simulink model "soc_opt5_compressed"  (R2026a)
settings: Solver=FixedStepDiscrete  StopTime=9  FixedStep=1
values from neighbouring files (symbols this model uses):
  compNet = s.bestNet    [build_simulink_model.m]    (also in save_slx.m; setup_and_open_slx.m; step2_simulink_sim.m)
libraries: dlconvfclib x2, dlsequencelib x2, dlactivationlib x1
Description:
  | SOC estimation: proj10_quant (neuronPCA 10%% + dlquantizer int8). 77.5%% Flash savings. MAE=9.50e-04 vs PyTorch. MATLAB R2026a.
settings Model: Creator=arkadiyturevskiy  LastModifiedBy=arkadiyturevskiy
settings HardwareCC: ProdLargestAtomicInteger=Long  ProdLargestAtomicFloat=Double  ProdHWDeviceType=ARM Compatible->ARM Cortex-M
settings RTWCC: SystemTargetFile=ert.tlc  PortableWordSizes=on  Description=Embedded Coder
settings ERTTargetCC: GenerateSampleERTMain=on

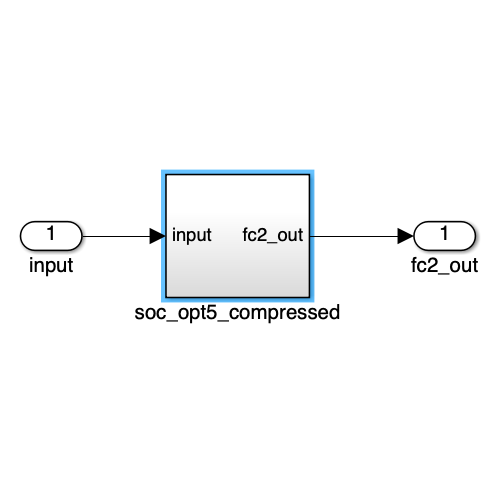
[thumbnail: Simulink's stored preview of the top-level diagram]
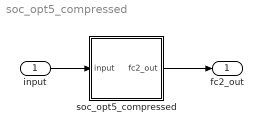
== system soc_opt5_compressed ==
  input : Inport  PortDimensions="[5  1]"
  soc_opt5_compressed : Subsystem
  fc2_out : Outport
  wires:
  soc_opt5_compressed/1(fc2_out) -> fc2_out/1
  input/1 -> soc_opt5_compressed/1(input)

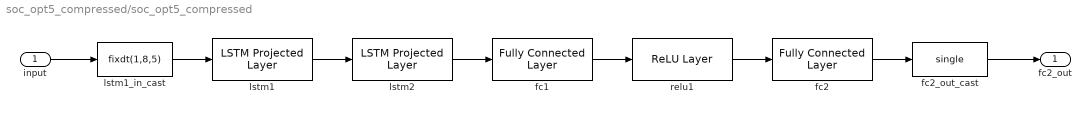
== system soc_opt5_compressed/soc_opt5_compressed ==
  input : Inport  PortDimensions="[5  1]"
  fc1 : dlconvfclib/Fully Connected Layer  Layer=compNet.Layers(4)  OutMin=[]  OutMax=[]  OutDataTypeStr=fixdt(1,8,7)  RndMeth=Nearest  SaturateOnIntegerOverflow=on  WeightsDataTypeStr=fixdt(1,8,10)  WeightsMin=[]  WeightsMax=[]  BiasDataTypeStr=fixdt(1,32,19)  BiasMin=[]  BiasMax=[]  AccumDataTypeStr=fixdt(1,32,19)  AccumMin=[]  AccumMax=[]  InternalRndMeth=Nearest  InternalSaturateOnIntegerOverflow=off  SampleTime=-1
      settings: DataFormat=C
  fc2 : dlconvfclib/Fully Connected Layer  Layer=compNet.Layers(6)  OutMin=[]  OutMax=[]  OutDataTypeStr=fixdt(1,32,17)  RndMeth=Nearest  WeightsDataTypeStr=fixdt(1,8,10)  WeightsMin=[]  WeightsMax=[]  BiasDataTypeStr=fixdt(1,32,17)  BiasMin=[]  BiasMax=[]  AccumDataTypeStr=fixdt(1,32,17)  AccumMin=[]  AccumMax=[]  InternalRndMeth=Nearest  InternalSaturateOnIntegerOverflow=off  SampleTime=-1
      settings: DataFormat=C
  fc2_out_cast : DataTypeConversion  OutDataTypeStr=single  SaturateOnIntegerOverflow=off  RndMeth=Floor
  lstm1 : dlsequencelib/LSTM Projected Layer  Layer=compNet.Layers(2)  Stateful=on  ApproximationMethod=Lookup  OutMin=[]  OutMax=[]  OutDataTypeStr=fixdt(1,8,8)  RndMeth=Nearest  SaturateOnIntegerOverflow=on  InputWeightsDataTypeStr=fixdt(1,8,9)  InputWeightsMin=[]  InputWeightsMax=[]  RecurrentWeightsDataTypeStr=fixdt(1,8,8)  RecurrentWeightsMin=[]  RecurrentWeightsMax=[]  BiasDataTypeStr=fixdt(1,32,19)  BiasMin=[]  BiasMax=[]  InputProjectorWeightsDataTypeStr=fixdt(1,8,7)  InputProjectorWeightsMin=[]  InputProjectorWeightsMax=[]  OutputProjectorWeightsDataTypeStr=fixdt(1,8,8)  OutputProjectorWeightsMin=[]  OutputProjectorWeightsMax=[]  InitialCellStateDataTypeStr=fixdt(1,16,15)  InitialCellStateMin=[]  InitialCellStateMax=[]  CellStateDataTypeStr=fixdt(1,16,15)  CellStateMin=[]  CellStateMax=[]  InitialHiddenStateDataTypeStr=fixdt(1,8,8)  InitialHiddenStateMin=[]  InitialHiddenStateMax=[]  HiddenStateDataTypeStr=fixdt(1,8,8)  HiddenStateMin=[]  HiddenStateMax=[]  InputWeightsMatrixMultiplyOutDataTypeStr=fixdt(1,32,19)  InputWeightsMatrixMultiplyOutMin=[]  InputWeightsMatrixMultiplyOutMax=[]  RecurrentWeightsMatrixMultiplyOutDataTypeStr=fixdt(1,32,19)  RecurrentWeightsMatrixMultiplyOutMin=[]  RecurrentWeightsMatrixMultiplyOutMax=[]  InputProjectorWeightsMatrixMultiplyOutDataTypeStr=fixdt(1,16,10)  InputProjectorWeightsMatrixMultiplyOutMin=[]  InputProjectorWeightsMatrixMultiplyOutMax=[]  OutputProjectorWeightsMatrixMultiplyOutDataTypeStr=fixdt(1,16,10)  OutputProjectorWeightsMatrixMultiplyOutMin=[]  OutputProjectorWeightsMatrixMultiplyOutMax=[]  LinearGateAccumDataTypeStr=fixdt(1,32,19)  LinearGateAddOutDataTypeStr=fixdt(1,16,12)  LinearGateAddOutMin=[]  LinearGateAddOutMax=[]  GateActivationOutDataTypeStr=fixdt(0,16,16)  GateActivationInputDataTypeStr=fixdt(1,16,11)  StateActivationOutDataTypeStr=fixdt(1,16,15)  StateActivationInputDataTypeStr=fixdt(1,16,12)  CellStateProductOutDataTypeStr=fixdt(1,32,15)  CellStateProductOutMin=[]  CellStateProductOutMax=[]  CellStateAccumDataTypeStr=fixdt(1,32,15)  SampleTime=-1
      settings: DataFormat=CT
  lstm1_in_cast : DataTypeConversion  OutDataTypeStr=fixdt(1,8,5)  RndMeth=Nearest
  lstm2 : dlsequencelib/LSTM Projected Layer  Layer=compNet.Layers(3)  Stateful=on  ApproximationMethod=Lookup  OutMin=[]  OutMax=[]  OutDataTypeStr=fixdt(1,8,9)  RndMeth=Nearest  SaturateOnIntegerOverflow=on  InputWeightsDataTypeStr=fixdt(1,8,8)  InputWeightsMin=[]  InputWeightsMax=[]  RecurrentWeightsDataTypeStr=fixdt(1,8,8)  RecurrentWeightsMin=[]  RecurrentWeightsMax=[]  BiasDataTypeStr=fixdt(1,32,19)  BiasMin=[]  BiasMax=[]  InputProjectorWeightsDataTypeStr=fixdt(1,8,8)  InputProjectorWeightsMin=[]  InputProjectorWeightsMax=[]  OutputProjectorWeightsDataTypeStr=fixdt(1,8,8)  OutputProjectorWeightsMin=[]  OutputProjectorWeightsMax=[]  InitialCellStateDataTypeStr=fixdt(1,16,16)  InitialCellStateMin=[]  InitialCellStateMax=[]  CellStateDataTypeStr=fixdt(1,16,16)  CellStateMin=[]  CellStateMax=[]  InitialHiddenStateDataTypeStr=fixdt(1,8,9)  InitialHiddenStateMin=[]  InitialHiddenStateMax=[]  HiddenStateDataTypeStr=fixdt(1,8,9)  HiddenStateMin=[]  HiddenStateMax=[]  InputWeightsMatrixMultiplyOutDataTypeStr=fixdt(1,32,19)  InputWeightsMatrixMultiplyOutMin=[]  InputWeightsMatrixMultiplyOutMax=[]  RecurrentWeightsMatrixMultiplyOutDataTypeStr=fixdt(1,32,19)  RecurrentWeightsMatrixMultiplyOutMin=[]  RecurrentWeightsMatrixMultiplyOutMax=[]  InputProjectorWeightsMatrixMultiplyOutDataTypeStr=fixdt(1,16,10)  InputProjectorWeightsMatrixMultiplyOutMin=[]  InputProjectorWeightsMatrixMultiplyOutMax=[]  OutputProjectorWeightsMatrixMultiplyOutDataTypeStr=fixdt(1,16,11)  OutputProjectorWeightsMatrixMultiplyOutMin=[]  OutputProjectorWeightsMatrixMultiplyOutMax=[]  LinearGateAccumDataTypeStr=fixdt(1,32,19)  LinearGateAddOutDataTypeStr=fixdt(1,16,12)  LinearGateAddOutMin=[]  LinearGateAddOutMax=[]  GateActivationOutDataTypeStr=fixdt(0,16,16)  GateActivationInputDataTypeStr=fixdt(1,16,11)  StateActivationOutDataTypeStr=fixdt(1,16,15)  StateActivationInputDataTypeStr=fixdt(1,16,12)  CellStateProductOutDataTypeStr=fixdt(1,32,16)  CellStateProductOutMin=[]  CellStateProductOutMax=[]  CellStateAccumDataTypeStr=fixdt(1,32,16)  SampleTime=-1
      settings: DataFormat=CT
  relu1 : dlactivationlib/ReLU Layer  OutMin=[]  OutMax=[]  OutDataTypeStr=fixdt(1,8,7)  SampleTime=-1
  fc2_out : Outport
  wires:
  fc2_out_cast/1 -> fc2_out/1
  fc2/1 -> fc2_out_cast/1
  lstm1_in_cast/1 -> lstm1/1
  lstm2/1 -> fc1/1
  input/1 -> lstm1_in_cast/1
  lstm1/1 -> lstm2/1
  relu1/1 -> fc2/1
  fc1/1 -> relu1/1
